simulink model "Efficency_Benchmarking"  (R2022b)
settings: Solver=VariableStepAuto  StartTime=0.0  StopTime=400  MaxStep=.01  RelTol=1e-3  AbsTol=1e-3
values from neighbouring files (symbols this model uses):
  Output_Torque = 100    [Dyno_Plotter.m]    (also in Efficency_Benchmark.m = Output_Torque_list(i); Pull_Data_Plotter.m = Pull(12,:))
libraries: fl_lib x10, nesl_utility x6, simulink x3, sdl_lib x2, sh_lib x1
settings Model: Creator=david  LastModifiedBy=david
settings SolverCC: AutoScaleAbsTol=off  AlgebraicLoopSolver=TrustRegion  MaxZcPerStep=1
settings DebuggingCC: UnconnectedInputMsg=warning  UnconnectedOutputMsg=warning  UnconnectedLineMsg=warning  SymbolicDimsDataTypeCodeGenerationDiagnostic=none  SFMachineParentedDataDiag=warning
settings ModelReferenceCC: EnableRefExpFcnMdlSchedulingChecks=on
settings SFSimCC: CustomCodeUndefinedFunction=UseInterfaceOnly
settings RTWCC: DLArmComputeVersion=19.05
settings SimscapeCC: SimscapeLogType=all  SimscapeLogSimulationStatistics=on  SimscapeLogDataHistory=10000

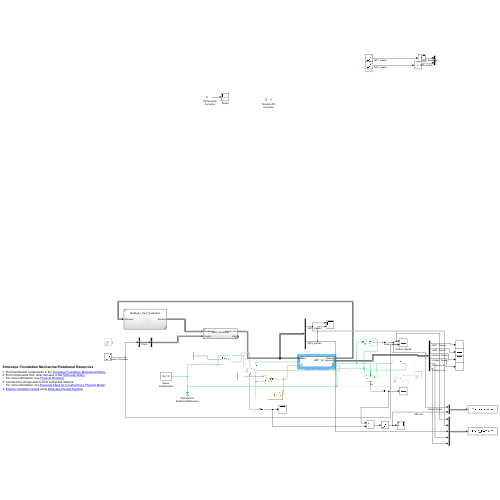
[thumbnail: Simulink's stored preview of the top-level diagram]
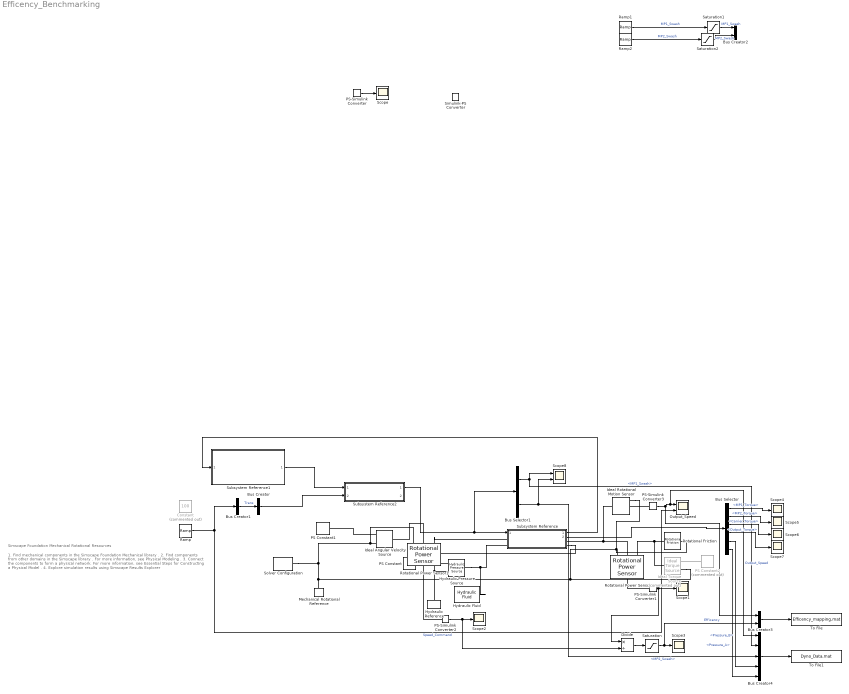
== system Efficency_Benchmarking ==
  note: 1. Find mechanical components in the Simscape Foundation Mechanical library .
      | 2. Find components from other domains in the Simscape library .
      | For more information, see Physical Modeling .
      | 3. Connect the components to form a physical network.
      | For more information, see Essential Steps for Constructing a Physical Model .
      | 4. Explore simulation results using Simscape Results Explorer
  note: Simscape Foundation Mechanical Rotational Resources
  Bus Creator : BusCreator  Inputs=1
  Bus Creator1 : BusCreator  Inputs=1
  Bus Creator2 : BusCreator  Inputs=2
  Bus Creator3 : BusCreator  Inputs=2
  Bus Creator4 : BusCreator  Inputs=5
  Bus Selector : BusSelector  OutputSignals=MP1_Torque,MP2_Torque,Carrier_Torque,Output_Torque,Pressure_B,Pressure_A
  Bus Selector1 : BusSelector  OutputSignals=MP1_Swash,MP2_Swash
  Constant : Constant  Commented=on  Value=100
  Divide : Product  Inputs=*/
  Hydraulic Fluid : sh_lib/Hydraulic Utilities/Hydraulic Fluid  SelFluid=15  SysTemp=60  TrapAir=0.005  ViscDerFactor=1  range_error=2
  Hydraulic Pressure Source : fl_lib/Hydraulic/Hydraulic Sources/Hydraulic Pressure Source
      settings: InternalSimscapePortConfiguration="{\"Bottom\":[],\"Left\":[{\"id\":\"P\",\"label\":\"P\",\"type\":\"foundation.hydraulic.hydraulic\"}],\"Right\":[{\"id\":\"S\",\"label\":\"S\",\"type\":\"input\"},{\"id\":\"T\",\"label\":\"T\",\"type\":\"foundation.hydraulic.hydraulic\"}],\"Top\":[]}"
  Hydraulic Reference : fl_lib/Hydraulic/Hydraulic Elements/Hydraulic Reference
  Ideal Angular Velocity Source : fl_lib/Mechanical/Mechanical Sources/Ideal Angular Velocity Source
  Ideal Rotational Motion Sensor : fl_lib/Mechanical/Mechanical Sensors/Ideal Rotational Motion Sensor  reference=foundation.enum.MeasurementReference.difference  acceleration_port=false  velocity_port=true  position_port=true  wrap_angle=false  offset=0 rad
  Ideal Torque Source : fl_lib/Mechanical/Mechanical Sources/Ideal Torque Source  Commented=on
  Mechanical Rotational Reference : fl_lib/Mechanical/Rotational Elements/Mechanical Rotational Reference
  Output_Speed : Scope  NumInputPorts=2
  PS Constant : fl_lib/Physical Signals/Sources/PS Constant  constant=150 psi
  PS Constant1 : fl_lib/Physical Signals/Sources/PS Constant  constant=Efficency_input_speed rpm
  PS Constant2 : fl_lib/Physical Signals/Sources/PS Constant  Commented=on  constant=Output_Torque ft*lb
  PS-Simulink Converter : nesl_utility/PS-Simulink Converter  PhysicalDomain=network_engine_domain  SubClassName=ps_output  LeftPortType=input  RightPortType=output  PseudoPeriodic=off  Frequencies=[]  VectorFormat=inherit  Unit=inherit  AffineConversion=off
  PS-Simulink Converter1 : nesl_utility/PS-Simulink Converter  PhysicalDomain=network_engine_domain  SubClassName=ps_output  LeftPortType=input  RightPortType=output  PseudoPeriodic=off  Frequencies=[]  VectorFormat=inherit  Unit=inherit  AffineConversion=off
  PS-Simulink Converter2 : nesl_utility/PS-Simulink Converter  PhysicalDomain=network_engine_domain  SubClassName=ps_output  LeftPortType=input  RightPortType=output  PseudoPeriodic=off  Frequencies=[]  VectorFormat=inherit  Unit=inherit  AffineConversion=off
  PS-Simulink Converter3 : nesl_utility/PS-Simulink Converter  PhysicalDomain=network_engine_domain  SubClassName=ps_output  LeftPortType=input  RightPortType=output  PseudoPeriodic=off  Frequencies=[]  VectorFormat=inherit  Unit=rpm  AffineConversion=off
  Ramp : simulink/Sources/Ramp  slope=7  start=0  InitialOutput=-300
  Ramp1 : simulink/Sources/Ramp  slope=-.01  start=0  InitialOutput=0
  Ramp2 : simulink/Sources/Ramp  slope=.01  start=100  InitialOutput=-1
  Rotational Friction : fl_lib/Mechanical/Rotational Elements/Rotational Friction  brkwy_trq=Output_Torque lbf*ft  brkwy_vel=0.1 rad/s  Col_trq=Output_Torque-.1 lbf*ft  visc_coef=0.001 N*m*s/rad  w_specify=off  w_priority=None  w=0 rad/s  w_nominal_specify=off  w_nominal_unit=rad/s  w_nominal_value=1  t_specify=off  t_priority=None  t=0 N*m  t_nominal_specify=off  t_nominal_unit=N*m  t_nominal_value=1
  Rotational Power Sensor : sdl_lib/Sensors/Rotational Power Sensor  measurement_type=sdl.enum.rotationalPowerSensorType.instantaneous  averaging_period=1 s  max_frequency=1000 Hz  max_speed=1000 rpm
      settings: InternalSimscapePortConfiguration="{\"Bottom\":[],\"Left\":[{\"id\":\"S\",\"label\":\"S\",\"type\":\"foundation.mechanical.rotational.rotational\"},{\"id\":\"R\",\"label\":\"R\",\"type\":\"foundation.mechanical.rotational.rotational\"},{\"id\":\"C\",\"label\":\"C\",\"type\":\"foundation.mechanical.rotational.rotational\"}],\"Right\":[{\"id\":\"P\",\"label\":\"P\",\"type\":\"output\"}],\"Top\":[]}"
  Rotational Power Sensor1 : sdl_lib/Sensors/Rotational Power Sensor  measurement_type=sdl.enum.rotationalPowerSensorType.instantaneous  averaging_period=1 s  max_frequency=1000 Hz  max_speed=1000 rpm
      settings: InternalSimscapePortConfiguration="{\"Bottom\":[],\"Left\":[{\"id\":\"S\",\"label\":\"S\",\"type\":\"foundation.mechanical.rotational.rotational\"},{\"id\":\"R\",\"label\":\"R\",\"type\":\"foundation.mechanical.rotational.rotational\"},{\"id\":\"C\",\"label\":\"C\",\"type\":\"foundation.mechanical.rotational.rotational\"}],\"Right\":[{\"id\":\"P\",\"label\":\"P\",\"type\":\"output\"}],\"Top\":[]}"
  Saturation : Saturate  UpperLimit=1  LowerLimit=-1
  Saturation1 : Saturate  UpperLimit=1  LowerLimit=-1
  Saturation2 : Saturate  UpperLimit=1  LowerLimit=-1
  Scope{,1..7} (8 alike) : Scope
  Scope8 : Scope  NumInputPorts=2
  Simulink-PS Converter : nesl_utility/Simulink-PS Converter  PhysicalDomain=network_engine_domain  SubClassName=ps_input  LeftPortType=input  RightPortType=output  PseudoPeriodic=off  Frequencies=[]  NoiseDistribution=none  NoiseParameters=[]  Unit=1  AffineConversion=off  FilteringAndDerivatives=provide  SimscapeFilterOrder=1  InputFilterTimeConstant=0.001  UdotUserProvided=0
  Solver Configuration : nesl_utility/Solver Configuration  PhysicalDomain=network_engine_domain  SubClassName=solver  LeftPortType=input  RightPortType=generic  Tones=[]  Harmonics=[]  SimulateNoise=off  Profile=off  UseLocalSampling=off  EnableSwitchedLinearOptims=on  FrequencyDomain=off  UseCCode=off  RelTol=0.001  AbsTol=1e-06  MinStep=1e-09  ToWorkspace=off  RevertToSquareIcSolve=off  NumHomotopyIterations=100  PhasorMode=off  PhasorModeNumHarmonics=1  ConsistencySolver=NEWTON_XTOL_AFTER_FTOL  IndexReductionMethod=DerivativeReplacement  DoDC=off  ResidualTolerance=1e-09  ConsistencyTolSource=GLOBAL  ConsistencyAbsTol=0.001  ConsistencyRelTol=0.001  ConsistencyTolFactor=0.001  UseLocalSolver=off  LocalSolverChoice=NE_BACKWARD_EULER_ADVANCER  ResolveIndetEquations=on  FunctionEvalNumThread=1  LocalSolverSampleTime=0.001  DoFixedCost=off  MaxNonlinIter=3  MaxModeIter=2  ComputeImpulses=off  ImpulseIterations=2  LinearAlgebra=auto  LinearAlgebraNumThread=0  EquationFormulation=NE_TIME_EF  DelaysMemoryBudget=1024  AutomaticFiltering=on  FilteringTimeConstant=0.001  PartitionStorageMethod=AS_NEEDED  PartitionMemoryBudget=1024  PartitionMethod=ROBUST
  Subsystem Reference : Subsystem  ReferencedSubsystem=HMT
      settings: PortSchema="{\"entries\":[{\"content\":{\"sides\":[{\"content\":{\"connectorIds\":[\"In1\",\"RConn1\",\"LConn2\"]},\"type\":\"ConnectorPlacement.EquallySpacedRectSide\",\"uuid\":\"fdedb491-33de-44d0-87bf-4d938b73adb2\"},{\"content\":{\"connectorIds\":[\"Out1\",\"Out2\",\"LConn1\",\"RConn2\"],\"side\":\"RIGHT\"},\"type\":\"ConnectorPlacement.EquallySpacedRectSide\",\"uuid\":\"846da588-6b34-4f0a-8826-c79aa7268cc7\"},{\"content\":{\"connectorIds\":[],\"side\":\"TOP\"},\"type\":\"ConnectorPlacement.EquallySpacedRectSide\",\"uuid\":\"12499447-05b1-4785-87b7-03b761060a74\"}]},\"type\":\"ConnectorPlacement.EquallySpacedConnector\",\"uuid\":\"53284d45-9163-442b-91da-45ee3b70adf9\"}],\"packageUris\":[\"http://schema.mathworks.com/mf0/Connector/R2020b\"],\"version\":\"1.0\"}"
  Subsystem Reference1 : Subsystem  ReferencedSubsystem=Multibody_Input_Calibration
  Subsystem Reference2 : Subsystem  ReferencedSubsystem=HMT_Controller
  To File : ToFile  Filename=Efficency_mapping.mat  MatrixName=Eff  SampleTime=.1
  To File1 : ToFile  Filename=Dyno_Data.mat  MatrixName=Dyno  SampleTime=.1
  wires:
  PS-Simulink Converter/1 -> Scope/1
  Subsystem Reference1/1 -> Subsystem Reference2/1
  Bus Creator/1 -> Subsystem Reference2/2
  Subsystem Reference/1 -> Subsystem Reference1/1
  PS-Simulink Converter1/1 -> Divide/1, Scope1/1
  Bus Creator1/1 -> Bus Creator/1  "Trans"
  PS-Simulink Converter2/1 -> Divide/2, Scope2/1
  Divide/1 -> Saturation/1
  Saturation/1 -> Bus Creator3/2, Scope3/1  "Efficency"
  Subsystem Reference/2 -> Bus Selector/1
  Bus Selector/1 -> Scope4/1  "<MP1_Torque>"
  Bus Selector/2 -> Scope5/1  "<MP2_Torque>"
  Bus Selector/3 -> Scope6/1  "<Carrier_Torque>"
  Bus Selector/4 -> Scope7/1  "<Output_Torque>"
  Bus Selector1/1 -> Bus Creator4/2, Scope8/1  "<MP1_Swash>"
  Bus Selector1/2 -> Bus Creator4/3, Scope8/2  "<MP2_Swash>"
  PS-Simulink Converter3/1 -> Bus Creator3/1, Bus Creator4/1, Output_Speed/1  "Output_Speed"
  Ramp/1 -> Bus Creator1/1, Output_Speed/2  "Speed_Command"
  Saturation1/1 -> Bus Creator2/1  "MP1_Swash"
  Saturation2/1 -> Bus Creator2/2  "MP2_Swash"
  Bus Creator3/1 -> To File/1
  Bus Creator4/1 -> To File1/1
  Bus Selector/5 -> Bus Creator4/4  "<Pressure_B>"
  Bus Selector/6 -> Bus Creator4/5  "<Pressure_A>"
  Ramp2/1 -> Saturation2/1  "MP2_Swash"
  Ramp1/1 -> Saturation1/1  "MP1_Swash"
  Subsystem Reference2/1 -> Bus Selector1/1, Subsystem Reference/1
  connections:
  Solver Configuration/RConn1 -- Rotational Power Sensor1/LConn3 -- Ideal Angular Velocity Source/RConn2 -- Ideal Torque Source/RConn2 -- Rotational Friction/RConn1 -- Ideal Rotational Motion Sensor/RConn1 -- Rotational Power Sensor/LConn3 -- Mechanical Rotational Reference/LConn1
  Hydraulic Pressure Source/RConn2 -- Hydraulic Reference/LConn1 -- Subsystem Reference/RConn2
  Hydraulic Pressure Source/LConn1 -- Hydraulic Fluid/RConn1 -- Subsystem Reference/LConn2
  Hydraulic Pressure Source/RConn1 -- PS Constant/RConn1
  Ideal Angular Velocity Source/RConn1 -- PS Constant1/RConn1
  Rotational Power Sensor/LConn2 -- Ideal Rotational Motion Sensor/LConn1 -- Subsystem Reference/LConn1
  Rotational Friction/LConn1 -- Ideal Torque Source/LConn1 -- Rotational Power Sensor/LConn1
  PS-Simulink Converter1/LConn1 -- Rotational Power Sensor/RConn1
  Rotational Power Sensor1/LConn1 -- Subsystem Reference/RConn1
  Rotational Power Sensor1/LConn2 -- Ideal Angular Velocity Source/LConn1
  PS-Simulink Converter2/LConn1 -- Rotational Power Sensor1/RConn1
  PS-Simulink Converter3/LConn1 -- Ideal Rotational Motion Sensor/RConn2
  PS Constant2/RConn1 -- Ideal Torque Source/RConn1
